simulink model "s0310"  (Simulink 6.0)
settings: Solver=ode3  SolverMode=SingleTasking  StartTime=0.0  StopTime=900  FixedStep=1  MaxStep=1  RelTol=1e-3  AbsTol=1e-6
values from neighbouring files (symbols this model uses):
  Kp = b01/a0*100    [m0221d.m]    (also in m0224.m = 3.3; m0225.m = 3.5; m0228.m = 1; m0232.m = 4)
  Kpz = -Ra/(c2*c3*Phi^2)    (= -0.025)    [m0310.m]
  ML0 = 0    [m0310.m]
  MLdach = 300    [m0310.m]
  T1 = 3*T1    (= 0.3)    [m0203.m]    (also in m0204.m = 0.1; m0205.m = 0.1; m0207.m = 0.1; m0221d.m = 1/a0)
  uA0 = 1/Kp*(wS-Kpz*ML0)    (= 0)    [m0310.m]
  uAdach = 40    [m0310.m]
settings Model: LastModifiedBy=Froriep
settings DataIOCC: LimitDataPoints=off  SaveOutput=off  SaveTime=off
settings OptimizationCC: BooleanDataType=off
settings DebuggingCC: SolverPrmCheckMsg=none
settings HardwareCC: TargetUnknown=on
settings GRTTargetCC: ModelReferenceCompliant=off  MatFileLogging=off

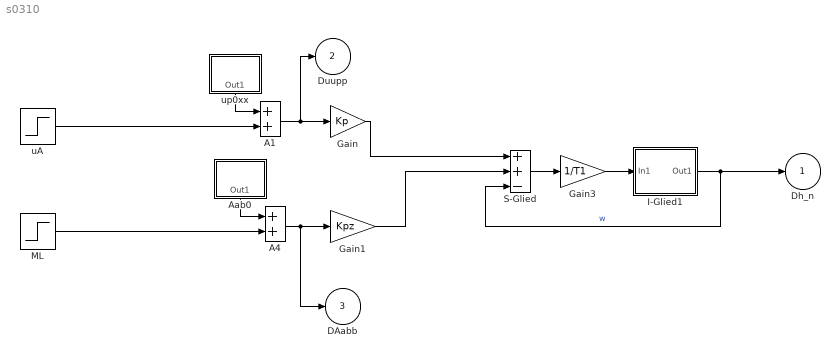
== system s0310 ==
  A1 : Sum  SaturateOnIntegerOverflow=on  InputSameDT=on
  A4 : Sum  SaturateOnIntegerOverflow=on  InputSameDT=on
  Aab0 : Subsystem  Orientation=down  mask(Konstante){Konst=ML0}
      mask prompts: Konst "Wert"
      mask help: Konstante
      mask Display: disp('ML0')
  Gain : Gain  Gain=Kp
  Gain1 : Gain  Gain=Kpz
  Gain3 : Gain  Gain=1/T1
  I-Glied1 : Subsystem  mask(I-Glied){@1=wS}
      mask prompts: @1 "Anfangswert"
      mask help: I-Glied
      mask init:
      | x0=@1;
      mask Display: disp('I-Glied')
  ML : Step  Time=2  After=MLdach  SampleTime=0
  S-Glied : Sum  Inputs=++-  SaturateOnIntegerOverflow=on  InputSameDT=on
  uA : Step  After=uAdach  SampleTime=0
  up0xx : Subsystem  Orientation=down  mask(Konstante){Konst=uA0}
      mask prompts: Konst "Wert"
      mask help: Konstante
      mask Display: disp('uA0')
  Dh_n : Outport
  Duupp : Outport  Port=2
  DAabb : Outport  Port=3
  wires:
  Aab0/1(Out1) -> A4/1
  up0xx/1(Out1) -> A1/1
  A1/1 -> Gain/1, Duupp/1
  A4/1 -> Gain1/1, DAabb/1
  uA/1 -> A1/2
  ML/1 -> A4/2
  I-Glied1/1(Out1) -> S-Glied/3, Dh_n/1  "w"
  Gain/1 -> S-Glied/1
  Gain1/1 -> S-Glied/2
  S-Glied/1 -> Gain3/1
  Gain3/1 -> I-Glied1/1(In1)

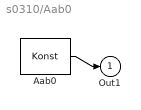
== system s0310/Aab0 ==
  Aab0 : Constant  Value=Konst
  Out1 : Outport
  wires:
  Aab0/1 -> Out1/1

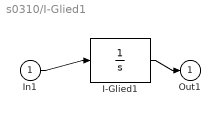
== system s0310/I-Glied1 ==
  In1 : Inport  Port=1  LatchInput=off
  I-Glied1 : Integrator  InitialCondition=x0
  Out1 : Outport
  wires:
  I-Glied1/1 -> Out1/1
  In1/1 -> I-Glied1/1

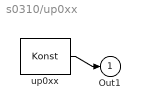
== system s0310/up0xx ==
  up0xx : Constant  Value=Konst
  Out1 : Outport
  wires:
  up0xx/1 -> Out1/1
